simulink model "NEWkrstic_example_1p3_wnoise"  (R2016b)
settings: Solver=ode45  StartTime=0.0  StopTime=100  RelTol=1e-3  EnableMultiTasking=on
libraries: simulink x1
settings Model: Creator=sbrunton  LastModifiedBy=sbrunton
settings DataIOCC: SaveFormat=Array  SignalLoggingSaveFormat=ModelDataLogs
settings OptimizationCC: ExpressionDepthLimit=2147483647  LifeSpan=inf
settings DebuggingCC: UnderspecifiedInitializationDetection=Classic  MergeDetectMultiDrivingBlocksExec=none  SolverPrmCheckMsg=warning  FcnCallInpInsideContextMsg=warning  StateNameClashWarn=warning  SFUnexpectedBacktrackingDiag=warning  SFNoUnconditionalDefaultTransitionDiag=warning  SFExecutionAtInitializationDiag=none
settings HardwareCC: ProdBitPerPointer=32  ProdBitPerSizeT=32  ProdBitPerPtrDiffT=32  ProdLargestAtomicFloat=None  ProdIntDivRoundTo=Undefined  ProdEndianess=Unspecified  ProdWordSize=32  ProdHWDeviceType=32-bit Generic
settings ModelReferenceCC: PropagateSignalLabelsOutOfModel=off
settings GRTTargetCC: TargetLangStandard=C89/C90 (ANSI)  CombineOutputUpdateFcns=off  GRTInterface=on
settings ConfigComp: CovMetricSettings=dw  CovHtmlReporting=on  CovSaveCumulativeToWorkspaceVar=on  CovSaveSingleToWorkspaceVar=on  CovExternalEMLEnable=off

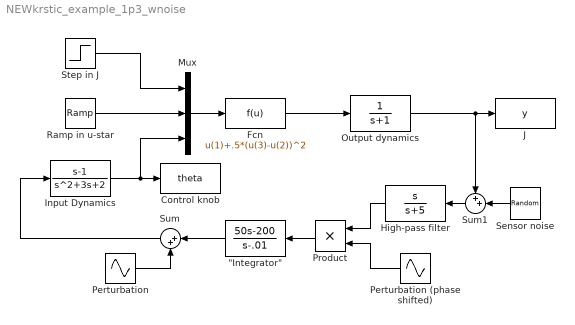
== system NEWkrstic_example_1p3_wnoise ==
  "\"Integrator\" " : TransferFcn  Numerator=[50 -200]  Denominator=[1 -.01]
  Control knob : ToWorkspace  VariableName=theta  SampleTime=-1
  Fcn : Fcn  Expr=u(1)+.5*(u(3)-u(2))^2
  High-pass filter : TransferFcn  Numerator=[1 0]  Denominator=[1 5]
  Input Dynamics : TransferFcn  Numerator=[1 -1]  Denominator=[1 3 2]
  J : ToWorkspace  VariableName=y  SampleTime=-1
  Mux : Mux  Inputs=3
  Output dynamics : TransferFcn  Denominator=[1 1]
  Perturbation : Sin  Amplitude=.05  Frequency=5  SampleTime=0
  Perturbation (phase shifted) : Sin  Frequency=5  Phase=.7955  SampleTime=0
  Product : Product  RndMeth=Zero
  Ramp in u-star : simulink/Sources/Ramp  slope=.001  start=0  X0=.01
  Sensor noise : UniformRandomNumber  Minimum=-.005  Maximum=.005  SampleTime=.001
  Step in J : Step  Time=10  After=.05  SampleTime=0
  Sum : Sum  Inputs=|++
  Sum1 : Sum  Inputs=++|
  wires:
  Output dynamics/1 -> J/1, Sum1/1
  Sum/1 -> Input Dynamics/1
  Ramp in u-star/1 -> Mux/2
  Step in J/1 -> Mux/1
  Input Dynamics/1 -> Mux/3, Control knob/1
  Mux/1 -> Fcn/1
  Fcn/1 -> Output dynamics/1
  High-pass filter/1 -> Product/1
  Perturbation (phase shifted)/1 -> Product/2
  Product/1 -> "\"Integrator\" "/1
  "\"Integrator\" "/1 -> Sum/1
  Perturbation/1 -> Sum/2
  Sum1/1 -> High-pass filter/1
  Sensor noise/1 -> Sum1/2
